simulink model "TST_SSpMon_Co"  (R2016b)
settings: Solver=FixedStepDiscrete  StartTime=0.0  StopTime=simTime  FixedStep=sampleTime  RelTol=1e-3
values from neighbouring files (symbols this model uses):
  testCase = 1    [initTST_SSpMon_Co_001.m]    (also in initTST_SSpMon_Co_002.m = 2)
libraries: simulink x3
settings Model: Creator=wolf072601  LastModifiedBy=wolf072601
settings DebuggingCC: SignalRangeChecking=error

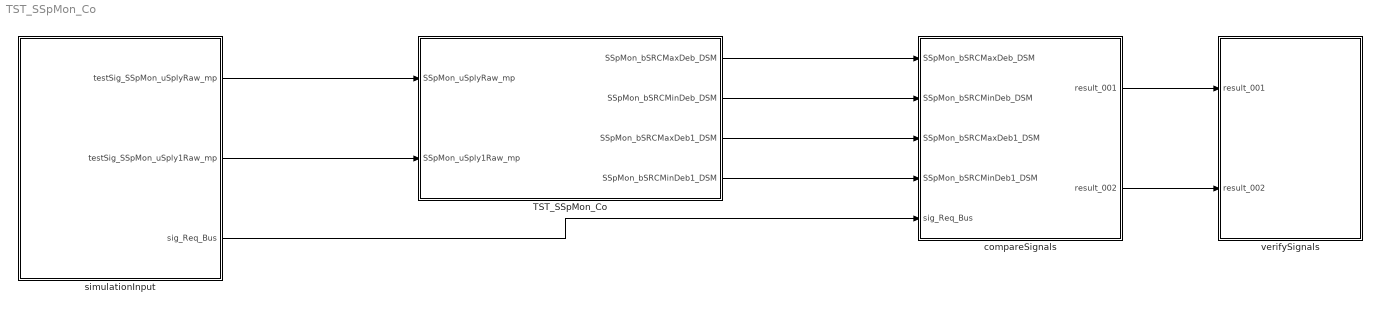
== system TST_SSpMon_Co ==
  TST_SSpMon_Co : Subsystem
  compareSignals : Subsystem
  simulationInput : Subsystem
  verifySignals : Subsystem
  wires:
  simulationInput/1(testSig_SSpMon_uSplyRaw_mp) -> TST_SSpMon_Co/1(SSpMon_uSplyRaw_mp)
  simulationInput/2(testSig_SSpMon_uSply1Raw_mp) -> TST_SSpMon_Co/2(SSpMon_uSply1Raw_mp)
  TST_SSpMon_Co/1(SSpMon_bSRCMaxDeb_DSM) -> compareSignals/1(SSpMon_bSRCMaxDeb_DSM)
  TST_SSpMon_Co/2(SSpMon_bSRCMinDeb_DSM) -> compareSignals/2(SSpMon_bSRCMinDeb_DSM)
  TST_SSpMon_Co/3(SSpMon_bSRCMaxDeb1_DSM) -> compareSignals/3(SSpMon_bSRCMaxDeb1_DSM)
  TST_SSpMon_Co/4(SSpMon_bSRCMinDeb1_DSM) -> compareSignals/4(SSpMon_bSRCMinDeb1_DSM)
  simulationInput/3(sig_Req_Bus) -> compareSignals/5(sig_Req_Bus)
  compareSignals/1(result_001) -> verifySignals/1(result_001)
  compareSignals/2(result_002) -> verifySignals/2(result_002)

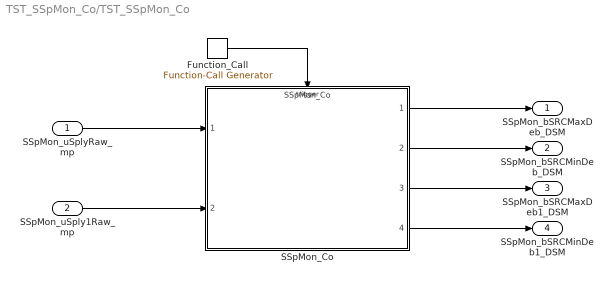
== system TST_SSpMon_Co/TST_SSpMon_Co ==
  SSpMon_uSplyRaw_mp : Inport
  SSpMon_uSply1Raw_mp : Inport  Port=2
  Function_Call : simulink/Ports & Subsystems/Function-Call Generator  sample_time=sampleTime  numberOfIterations=1
  SSpMon_Co : ModelReference  ModelNameDialog=SSpMon_Co  ModelReferenceVersion=1.7  TriggerPortName=function  TriggerPortTriggerType=function-call  TriggerPortStatesWhenEnabling=held
  SSpMon_bSRCMaxDeb_DSM : Outport
  SSpMon_bSRCMinDeb_DSM : Outport  Port=2
  SSpMon_bSRCMaxDeb1_DSM : Outport  Port=3
  SSpMon_bSRCMinDeb1_DSM : Outport  Port=4
  wires:
  Function_Call/1 -> SSpMon_Co/Trigger
  SSpMon_uSplyRaw_mp/1 -> SSpMon_Co/1
  SSpMon_uSply1Raw_mp/1 -> SSpMon_Co/2
  SSpMon_Co/1 -> SSpMon_bSRCMaxDeb_DSM/1
  SSpMon_Co/2 -> SSpMon_bSRCMinDeb_DSM/1
  SSpMon_Co/3 -> SSpMon_bSRCMaxDeb1_DSM/1
  SSpMon_Co/4 -> SSpMon_bSRCMinDeb1_DSM/1

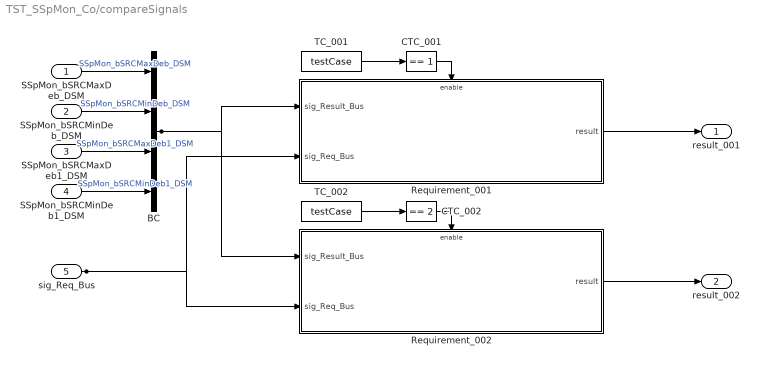
== system TST_SSpMon_Co/compareSignals ==
  SSpMon_bSRCMaxDeb_DSM : Inport
  SSpMon_bSRCMinDeb_DSM : Inport  Port=2
  SSpMon_bSRCMaxDeb1_DSM : Inport  Port=3
  SSpMon_bSRCMinDeb1_DSM : Inport  Port=4
  sig_Req_Bus : Inport  Port=5
  BC : BusCreator  Inputs=4
  CTC_001 : simulink/Logic and Bit Operations/Compare To Constant  relop===  const=1  OutDataTypeStr=boolean
  CTC_002 : simulink/Logic and Bit Operations/Compare To Constant  relop===  const=2  OutDataTypeStr=boolean
  Requirement_001 : Subsystem
  Requirement_002 : Subsystem
  TC_001 : Constant  Value=testCase
  TC_002 : Constant  Value=testCase
  result_001 : Outport
  result_002 : Outport  Port=2
  wires:
  SSpMon_bSRCMaxDeb_DSM/1 -> BC/1  "SSpMon_bSRCMaxDeb_DSM"
  SSpMon_bSRCMinDeb_DSM/1 -> BC/2  "SSpMon_bSRCMinDeb_DSM"
  SSpMon_bSRCMaxDeb1_DSM/1 -> BC/3  "SSpMon_bSRCMaxDeb1_DSM"
  SSpMon_bSRCMinDeb1_DSM/1 -> BC/4  "SSpMon_bSRCMinDeb1_DSM"
  TC_001/1 -> CTC_001/1
  CTC_001/1 -> Requirement_001/Enable
  sig_Req_Bus/1 -> Requirement_001/2(sig_Req_Bus), Requirement_002/2(sig_Req_Bus)
  BC/1 -> Requirement_001/1(sig_Result_Bus), Requirement_002/1(sig_Result_Bus)
  Requirement_001/1(result) -> result_001/1
  TC_002/1 -> CTC_002/1
  CTC_002/1 -> Requirement_002/Enable
  Requirement_002/1(result) -> result_002/1

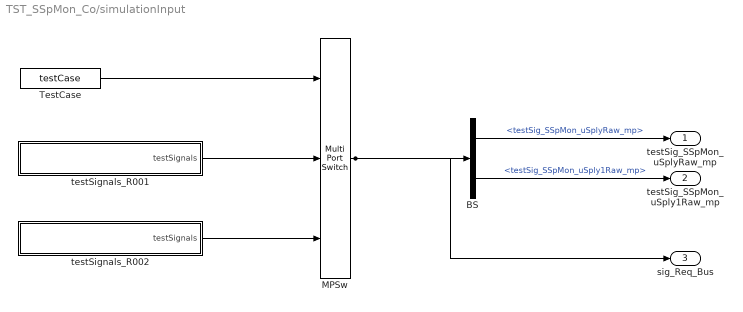
== system TST_SSpMon_Co/simulationInput ==
  BS : BusSelector  OutputSignals=testSig_SSpMon_uSplyRaw_mp,testSig_SSpMon_uSply1Raw_mp
  MPSw : MultiPortSwitch  Inputs=2  SaturateOnIntegerOverflow=on  InputSameDT=on
  TestCase : Constant  Value=testCase
  testSignals_R001 : Subsystem
  testSignals_R002 : Subsystem
  testSig_SSpMon_uSplyRaw_mp : Outport
  testSig_SSpMon_uSply1Raw_mp : Outport  Port=2
  sig_Req_Bus : Outport  Port=3
  wires:
  BS/1 -> testSig_SSpMon_uSplyRaw_mp/1  "<testSig_SSpMon_uSplyRaw_mp>"
  BS/2 -> testSig_SSpMon_uSply1Raw_mp/1  "<testSig_SSpMon_uSply1Raw_mp>"
  MPSw/1 -> BS/1, sig_Req_Bus/1
  TestCase/1 -> MPSw/1
  testSignals_R001/1(testSignals) -> MPSw/2
  testSignals_R002/1(testSignals) -> MPSw/3

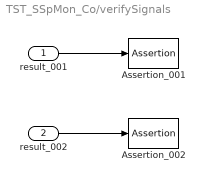
== system TST_SSpMon_Co/verifySignals ==
  result_001 : Inport
  result_002 : Inport  Port=2
  Assertion_001 : Assertion  Enabled=off
  Assertion_002 : Assertion  Enabled=off
  wires:
  result_001/1 -> Assertion_001/1
  result_002/1 -> Assertion_002/1

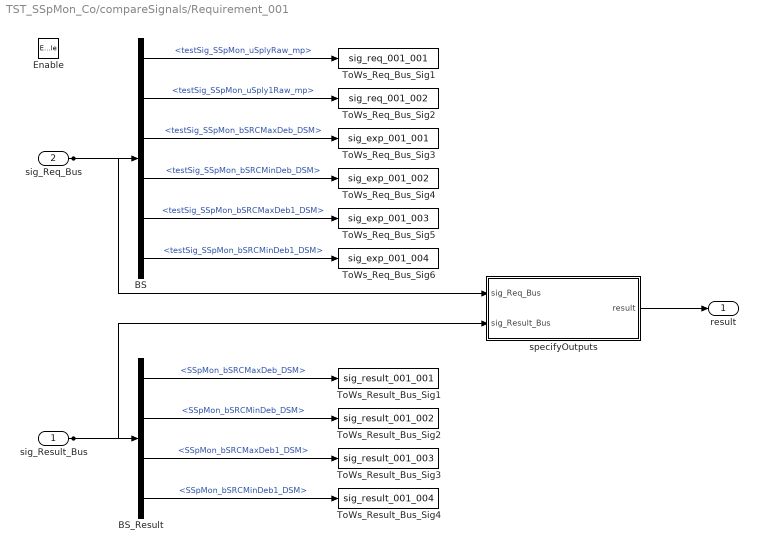
== system TST_SSpMon_Co/compareSignals/Requirement_001 ==
  sig_Result_Bus : Inport
  sig_Req_Bus : Inport  Port=2
  Enable : EnablePort
  BS : BusSelector  OutputSignals=testSig_SSpMon_uSplyRaw_mp,testSig_SSpMon_uSply1Raw_mp,testSig_SSpMon_bSRCMaxDeb_DSM,testSig_SSpMon_bSRCMinDeb_DSM,testSig_SSpMon_bSRCMaxDeb1_DSM,testSig_SSpMon_bSRCMinDeb1_DSM
  BS_Result : BusSelector  OutputSignals=SSpMon_bSRCMaxDeb_DSM,SSpMon_bSRCMinDeb_DSM,SSpMon_bSRCMaxDeb1_DSM,SSpMon_bSRCMinDeb1_DSM
  ToWs_Req_Bus_Sig1 : ToWorkspace  VariableName=sig_req_001_001  SaveFormat=Structure With Time
  ToWs_Req_Bus_Sig2 : ToWorkspace  VariableName=sig_req_001_002  SaveFormat=Structure With Time
  ToWs_Req_Bus_Sig3 : ToWorkspace  VariableName=sig_exp_001_001  SaveFormat=Structure With Time
  ToWs_Req_Bus_Sig4 : ToWorkspace  VariableName=sig_exp_001_002  SaveFormat=Structure With Time
  ToWs_Req_Bus_Sig5 : ToWorkspace  VariableName=sig_exp_001_003  SaveFormat=Structure With Time
  ToWs_Req_Bus_Sig6 : ToWorkspace  VariableName=sig_exp_001_004  SaveFormat=Structure With Time
  ToWs_Result_Bus_Sig1 : ToWorkspace  VariableName=sig_result_001_001  SaveFormat=Structure With Time
  ToWs_Result_Bus_Sig2 : ToWorkspace  VariableName=sig_result_001_002  SaveFormat=Structure With Time
  ToWs_Result_Bus_Sig3 : ToWorkspace  VariableName=sig_result_001_003  SaveFormat=Structure With Time
  ToWs_Result_Bus_Sig4 : ToWorkspace  VariableName=sig_result_001_004  SaveFormat=Structure With Time
  specifyOutputs : Subsystem
  result : Outport
  wires:
  sig_Req_Bus/1 -> BS/1, specifyOutputs/1(sig_Req_Bus)
  BS/1 -> ToWs_Req_Bus_Sig1/1  "<testSig_SSpMon_uSplyRaw_mp>"
  BS/2 -> ToWs_Req_Bus_Sig2/1  "<testSig_SSpMon_uSply1Raw_mp>"
  BS/3 -> ToWs_Req_Bus_Sig3/1  "<testSig_SSpMon_bSRCMaxDeb_DSM>"
  BS/4 -> ToWs_Req_Bus_Sig4/1  "<testSig_SSpMon_bSRCMinDeb_DSM>"
  BS/5 -> ToWs_Req_Bus_Sig5/1  "<testSig_SSpMon_bSRCMaxDeb1_DSM>"
  BS/6 -> ToWs_Req_Bus_Sig6/1  "<testSig_SSpMon_bSRCMinDeb1_DSM>"
  sig_Result_Bus/1 -> BS_Result/1, specifyOutputs/2(sig_Result_Bus)
  BS_Result/1 -> ToWs_Result_Bus_Sig1/1  "<SSpMon_bSRCMaxDeb_DSM>"
  BS_Result/2 -> ToWs_Result_Bus_Sig2/1  "<SSpMon_bSRCMinDeb_DSM>"
  BS_Result/3 -> ToWs_Result_Bus_Sig3/1  "<SSpMon_bSRCMaxDeb1_DSM>"
  BS_Result/4 -> ToWs_Result_Bus_Sig4/1  "<SSpMon_bSRCMinDeb1_DSM>"
  specifyOutputs/1(result) -> result/1

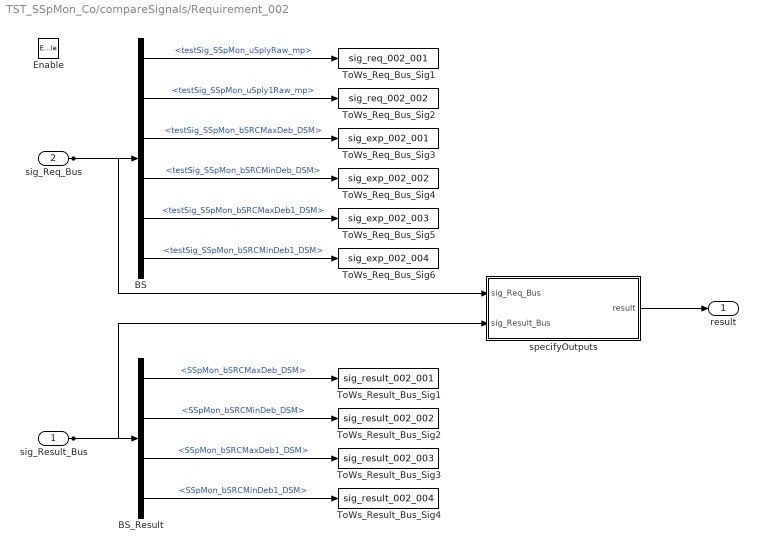
== system TST_SSpMon_Co/compareSignals/Requirement_002 ==
  sig_Result_Bus : Inport
  sig_Req_Bus : Inport  Port=2
  Enable : EnablePort
  BS : BusSelector  OutputSignals=testSig_SSpMon_uSplyRaw_mp,testSig_SSpMon_uSply1Raw_mp,testSig_SSpMon_bSRCMaxDeb_DSM,testSig_SSpMon_bSRCMinDeb_DSM,testSig_SSpMon_bSRCMaxDeb1_DSM,testSig_SSpMon_bSRCMinDeb1_DSM
  BS_Result : BusSelector  OutputSignals=SSpMon_bSRCMaxDeb_DSM,SSpMon_bSRCMinDeb_DSM,SSpMon_bSRCMaxDeb1_DSM,SSpMon_bSRCMinDeb1_DSM
  ToWs_Req_Bus_Sig1 : ToWorkspace  VariableName=sig_req_002_001  SaveFormat=Structure With Time
  ToWs_Req_Bus_Sig2 : ToWorkspace  VariableName=sig_req_002_002  SaveFormat=Structure With Time
  ToWs_Req_Bus_Sig3 : ToWorkspace  VariableName=sig_exp_002_001  SaveFormat=Structure With Time
  ToWs_Req_Bus_Sig4 : ToWorkspace  VariableName=sig_exp_002_002  SaveFormat=Structure With Time
  ToWs_Req_Bus_Sig5 : ToWorkspace  VariableName=sig_exp_002_003  SaveFormat=Structure With Time
  ToWs_Req_Bus_Sig6 : ToWorkspace  VariableName=sig_exp_002_004  SaveFormat=Structure With Time
  ToWs_Result_Bus_Sig1 : ToWorkspace  VariableName=sig_result_002_001  SaveFormat=Structure With Time
  ToWs_Result_Bus_Sig2 : ToWorkspace  VariableName=sig_result_002_002  SaveFormat=Structure With Time
  ToWs_Result_Bus_Sig3 : ToWorkspace  VariableName=sig_result_002_003  SaveFormat=Structure With Time
  ToWs_Result_Bus_Sig4 : ToWorkspace  VariableName=sig_result_002_004  SaveFormat=Structure With Time
  specifyOutputs : Subsystem
  result : Outport
  wires:
  sig_Req_Bus/1 -> BS/1, specifyOutputs/1(sig_Req_Bus)
  BS/1 -> ToWs_Req_Bus_Sig1/1  "<testSig_SSpMon_uSplyRaw_mp>"
  BS/2 -> ToWs_Req_Bus_Sig2/1  "<testSig_SSpMon_uSply1Raw_mp>"
  BS/3 -> ToWs_Req_Bus_Sig3/1  "<testSig_SSpMon_bSRCMaxDeb_DSM>"
  BS/4 -> ToWs_Req_Bus_Sig4/1  "<testSig_SSpMon_bSRCMinDeb_DSM>"
  BS/5 -> ToWs_Req_Bus_Sig5/1  "<testSig_SSpMon_bSRCMaxDeb1_DSM>"
  BS/6 -> ToWs_Req_Bus_Sig6/1  "<testSig_SSpMon_bSRCMinDeb1_DSM>"
  sig_Result_Bus/1 -> BS_Result/1, specifyOutputs/2(sig_Result_Bus)
  BS_Result/1 -> ToWs_Result_Bus_Sig1/1  "<SSpMon_bSRCMaxDeb_DSM>"
  BS_Result/2 -> ToWs_Result_Bus_Sig2/1  "<SSpMon_bSRCMinDeb_DSM>"
  BS_Result/3 -> ToWs_Result_Bus_Sig3/1  "<SSpMon_bSRCMaxDeb1_DSM>"
  BS_Result/4 -> ToWs_Result_Bus_Sig4/1  "<SSpMon_bSRCMinDeb1_DSM>"
  specifyOutputs/1(result) -> result/1

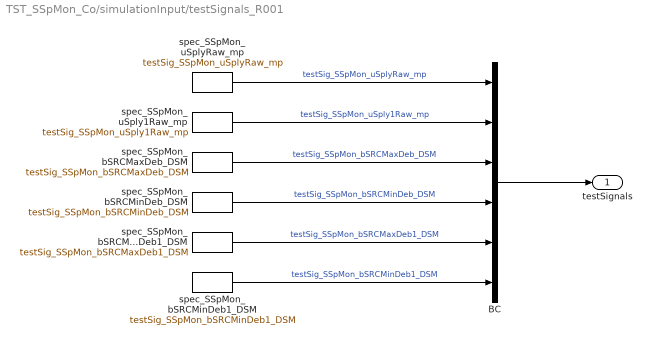
== system TST_SSpMon_Co/simulationInput/testSignals_R001 ==
  BC : BusCreator  Inputs=6
  spec_SSpMon_bSRCMaxDeb1_DSM : FromWorkspace  VariableName=testSig_SSpMon_bSRCMaxDeb1_DSM  Interpolate=off  OutputAfterFinalValue=Holding final value
  spec_SSpMon_bSRCMaxDeb_DSM : FromWorkspace  VariableName=testSig_SSpMon_bSRCMaxDeb_DSM  Interpolate=off  OutputAfterFinalValue=Holding final value
  spec_SSpMon_bSRCMinDeb1_DSM : FromWorkspace  VariableName=testSig_SSpMon_bSRCMinDeb1_DSM  Interpolate=off  OutputAfterFinalValue=Holding final value
  spec_SSpMon_bSRCMinDeb_DSM : FromWorkspace  VariableName=testSig_SSpMon_bSRCMinDeb_DSM  Interpolate=off  OutputAfterFinalValue=Holding final value
  spec_SSpMon_uSply1Raw_mp : FromWorkspace  VariableName=testSig_SSpMon_uSply1Raw_mp  Interpolate=off  OutputAfterFinalValue=Holding final value
  spec_SSpMon_uSplyRaw_mp : FromWorkspace  VariableName=testSig_SSpMon_uSplyRaw_mp  Interpolate=off  OutputAfterFinalValue=Holding final value
  testSignals : Outport
  wires:
  BC/1 -> testSignals/1
  spec_SSpMon_uSplyRaw_mp/1 -> BC/1  "testSig_SSpMon_uSplyRaw_mp"
  spec_SSpMon_uSply1Raw_mp/1 -> BC/2  "testSig_SSpMon_uSply1Raw_mp"
  spec_SSpMon_bSRCMaxDeb_DSM/1 -> BC/3  "testSig_SSpMon_bSRCMaxDeb_DSM"
  spec_SSpMon_bSRCMinDeb_DSM/1 -> BC/4  "testSig_SSpMon_bSRCMinDeb_DSM"
  spec_SSpMon_bSRCMaxDeb1_DSM/1 -> BC/5  "testSig_SSpMon_bSRCMaxDeb1_DSM"
  spec_SSpMon_bSRCMinDeb1_DSM/1 -> BC/6  "testSig_SSpMon_bSRCMinDeb1_DSM"

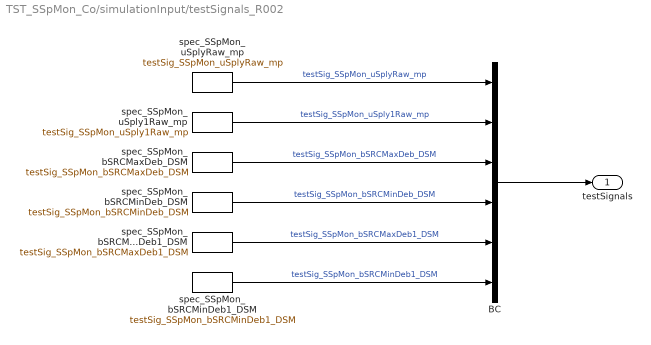
== system TST_SSpMon_Co/simulationInput/testSignals_R002 ==
  BC : BusCreator  Inputs=6
  spec_SSpMon_bSRCMaxDeb1_DSM : FromWorkspace  VariableName=testSig_SSpMon_bSRCMaxDeb1_DSM  Interpolate=off  OutputAfterFinalValue=Holding final value
  spec_SSpMon_bSRCMaxDeb_DSM : FromWorkspace  VariableName=testSig_SSpMon_bSRCMaxDeb_DSM  Interpolate=off  OutputAfterFinalValue=Holding final value
  spec_SSpMon_bSRCMinDeb1_DSM : FromWorkspace  VariableName=testSig_SSpMon_bSRCMinDeb1_DSM  Interpolate=off  OutputAfterFinalValue=Holding final value
  spec_SSpMon_bSRCMinDeb_DSM : FromWorkspace  VariableName=testSig_SSpMon_bSRCMinDeb_DSM  Interpolate=off  OutputAfterFinalValue=Holding final value
  spec_SSpMon_uSply1Raw_mp : FromWorkspace  VariableName=testSig_SSpMon_uSply1Raw_mp  Interpolate=off  OutputAfterFinalValue=Holding final value
  spec_SSpMon_uSplyRaw_mp : FromWorkspace  VariableName=testSig_SSpMon_uSplyRaw_mp  Interpolate=off  OutputAfterFinalValue=Holding final value
  testSignals : Outport
  wires:
  BC/1 -> testSignals/1
  spec_SSpMon_uSplyRaw_mp/1 -> BC/1  "testSig_SSpMon_uSplyRaw_mp"
  spec_SSpMon_uSply1Raw_mp/1 -> BC/2  "testSig_SSpMon_uSply1Raw_mp"
  spec_SSpMon_bSRCMaxDeb_DSM/1 -> BC/3  "testSig_SSpMon_bSRCMaxDeb_DSM"
  spec_SSpMon_bSRCMinDeb_DSM/1 -> BC/4  "testSig_SSpMon_bSRCMinDeb_DSM"
  spec_SSpMon_bSRCMaxDeb1_DSM/1 -> BC/5  "testSig_SSpMon_bSRCMaxDeb1_DSM"
  spec_SSpMon_bSRCMinDeb1_DSM/1 -> BC/6  "testSig_SSpMon_bSRCMinDeb1_DSM"

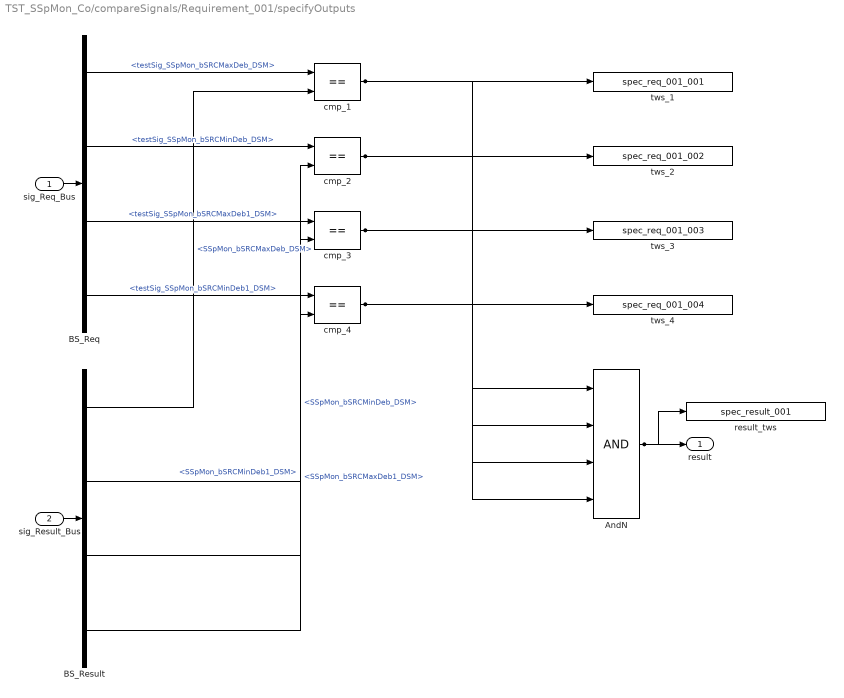
== system TST_SSpMon_Co/compareSignals/Requirement_001/specifyOutputs ==
  sig_Req_Bus : Inport
  sig_Result_Bus : Inport  Port=2
  AndN : Logic  Inputs=4
  BS_Req : BusSelector  OutputSignals=testSig_SSpMon_bSRCMaxDeb_DSM,testSig_SSpMon_bSRCMinDeb_DSM,testSig_SSpMon_bSRCMaxDeb1_DSM,testSig_SSpMon_bSRCMinDeb1_DSM
  BS_Result : BusSelector  OutputSignals=SSpMon_bSRCMaxDeb_DSM,SSpMon_bSRCMinDeb_DSM,SSpMon_bSRCMaxDeb1_DSM,SSpMon_bSRCMinDeb1_DSM
  cmp_{1..4} (4 alike) : RelationalOperator  Operator===  RndMeth=Nearest  InputSameDT=on
  result_tws : ToWorkspace  VariableName=spec_result_001
  tws_1 : ToWorkspace  VariableName=spec_req_001_001
  tws_2 : ToWorkspace  VariableName=spec_req_001_002
  tws_3 : ToWorkspace  VariableName=spec_req_001_003
  tws_4 : ToWorkspace  VariableName=spec_req_001_004
  result : Outport
  wires:
  sig_Req_Bus/1 -> BS_Req/1
  sig_Result_Bus/1 -> BS_Result/1
  AndN/1 -> result/1, result_tws/1
  BS_Req/1 -> cmp_1/1  "<testSig_SSpMon_bSRCMaxDeb_DSM>"
  BS_Result/1 -> cmp_1/2  "<SSpMon_bSRCMaxDeb_DSM>"
  cmp_1/1 -> tws_1/1, AndN/1
  BS_Req/2 -> cmp_2/1  "<testSig_SSpMon_bSRCMinDeb_DSM>"
  BS_Result/2 -> cmp_2/2  "<SSpMon_bSRCMinDeb_DSM>"
  cmp_2/1 -> tws_2/1, AndN/2
  BS_Req/3 -> cmp_3/1  "<testSig_SSpMon_bSRCMaxDeb1_DSM>"
  BS_Result/3 -> cmp_3/2  "<SSpMon_bSRCMaxDeb1_DSM>"
  cmp_3/1 -> tws_3/1, AndN/3
  BS_Req/4 -> cmp_4/1  "<testSig_SSpMon_bSRCMinDeb1_DSM>"
  BS_Result/4 -> cmp_4/2  "<SSpMon_bSRCMinDeb1_DSM>"
  cmp_4/1 -> tws_4/1, AndN/4

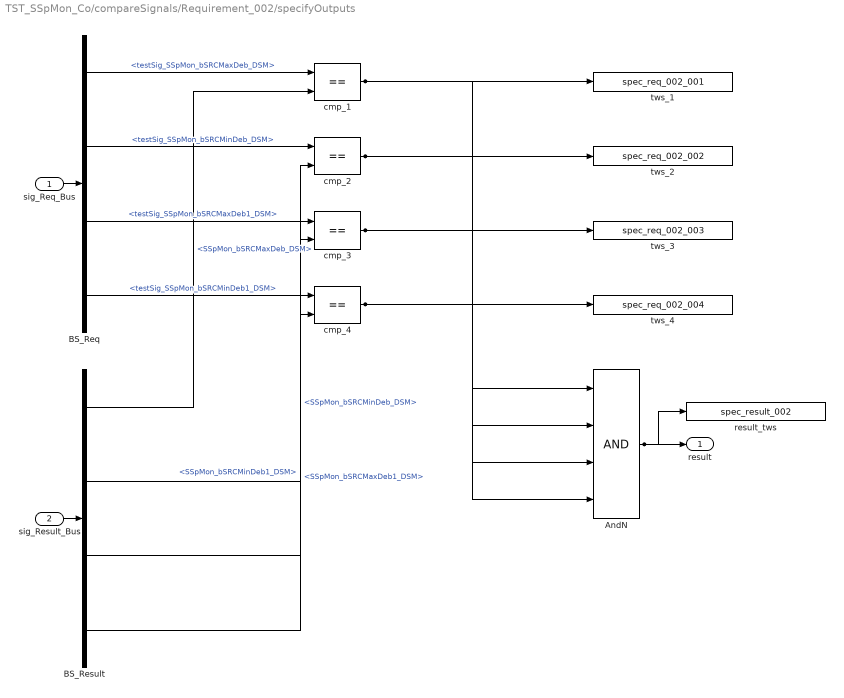
== system TST_SSpMon_Co/compareSignals/Requirement_002/specifyOutputs ==
  sig_Req_Bus : Inport
  sig_Result_Bus : Inport  Port=2
  AndN : Logic  Inputs=4
  BS_Req : BusSelector  OutputSignals=testSig_SSpMon_bSRCMaxDeb_DSM,testSig_SSpMon_bSRCMinDeb_DSM,testSig_SSpMon_bSRCMaxDeb1_DSM,testSig_SSpMon_bSRCMinDeb1_DSM
  BS_Result : BusSelector  OutputSignals=SSpMon_bSRCMaxDeb_DSM,SSpMon_bSRCMinDeb_DSM,SSpMon_bSRCMaxDeb1_DSM,SSpMon_bSRCMinDeb1_DSM
  cmp_{1..4} (4 alike) : RelationalOperator  Operator===  RndMeth=Nearest  InputSameDT=on
  result_tws : ToWorkspace  VariableName=spec_result_002
  tws_1 : ToWorkspace  VariableName=spec_req_002_001
  tws_2 : ToWorkspace  VariableName=spec_req_002_002
  tws_3 : ToWorkspace  VariableName=spec_req_002_003
  tws_4 : ToWorkspace  VariableName=spec_req_002_004
  result : Outport
  wires:
  sig_Req_Bus/1 -> BS_Req/1
  sig_Result_Bus/1 -> BS_Result/1
  AndN/1 -> result/1, result_tws/1
  BS_Req/1 -> cmp_1/1  "<testSig_SSpMon_bSRCMaxDeb_DSM>"
  BS_Result/1 -> cmp_1/2  "<SSpMon_bSRCMaxDeb_DSM>"
  cmp_1/1 -> tws_1/1, AndN/1
  BS_Req/2 -> cmp_2/1  "<testSig_SSpMon_bSRCMinDeb_DSM>"
  BS_Result/2 -> cmp_2/2  "<SSpMon_bSRCMinDeb_DSM>"
  cmp_2/1 -> tws_2/1, AndN/2
  BS_Req/3 -> cmp_3/1  "<testSig_SSpMon_bSRCMaxDeb1_DSM>"
  BS_Result/3 -> cmp_3/2  "<SSpMon_bSRCMaxDeb1_DSM>"
  cmp_3/1 -> tws_3/1, AndN/3
  BS_Req/4 -> cmp_4/1  "<testSig_SSpMon_bSRCMinDeb1_DSM>"
  BS_Result/4 -> cmp_4/2  "<SSpMon_bSRCMinDeb1_DSM>"
  cmp_4/1 -> tws_4/1, AndN/4
